simulink model "CPUTask"  (R2022b)
settings: Solver=FixedStepDiscrete  StartTime=0.0  StopTime=10.0  FixedStep=1  RelTol=1e-3
libraries: simulink x5
settings Model: Creator=sadamu  LastModifiedBy=sadamu
settings SolverCC: AlgebraicLoopSolver=TrustRegion
settings DataIOCC: ExternalInput=externalinputdata
settings OptimizationCC: DefaultParameterBehavior=Inlined  BufferReuse=off  GlobalBufferReuse=off  EnableMemcpy=off  PassReuseOutputArgsAs=Individual arguments  OptimizeDataStoreBuffers=off  BusAssignmentInplaceUpdate=off  OptimizationLevel=level0  OptimizationPriority=Speed  EfficientTunableParamExpr=on
settings DebuggingCC: ParameterTunabilityLossMsg=error  UnconnectedInputMsg=warning  UnconnectedOutputMsg=warning  UnconnectedLineMsg=warning  SFMachineParentedDataDiag=warning
settings ModelReferenceCC: EnableRefExpFcnMdlSchedulingChecks=on
settings SFSimCC: MATLABDynamicMemAlloc=off
settings RTWCC: Description=Embedded Coder  SystemTargetFile=ert.tlc  GenCodeOnly=on  TemplateMakefile=ert_default_tmf
settings CodeAppCC: GenerateComments=off  IgnoreCustomStorageClasses=off  OperatorAnnotations=on  SimulinkDataObjDesc=on  SFDataObjDesc=on  SimulinkBlockComments=off
settings ERTTargetCC: TargetLangStandard=C99 (ISO)  GenerateSampleERTMain=on  SuppressErrorStatus=on  CodeInterfacePackaging=Reusable function  InlinedParameterPlacement=NonHierarchical  MultiInstanceErrorCode=None  ERTCustomFileTemplate=example_file_process.tlc  ConvertIfToSwitch=off
settings ConfigComp: DVMaxProcessTime=3600  DVMaxTestCaseSteps=30  DVTestSuiteOptimization=Auto  DVDetectOutOfBounds=on  DVProvingStrategy=FindViolation  DVMaxViolationSteps=200000  DVModelReferenceHarness=on

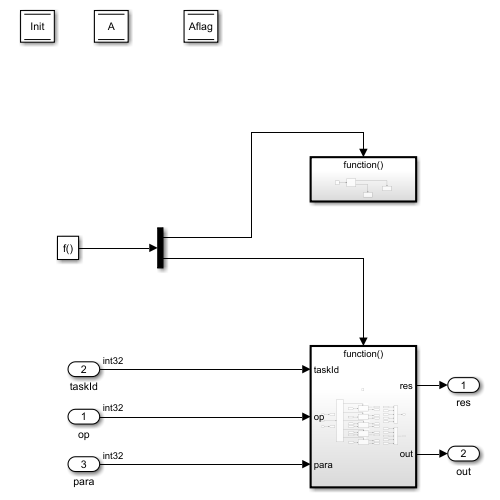
[thumbnail: Simulink's stored preview of the top-level diagram]
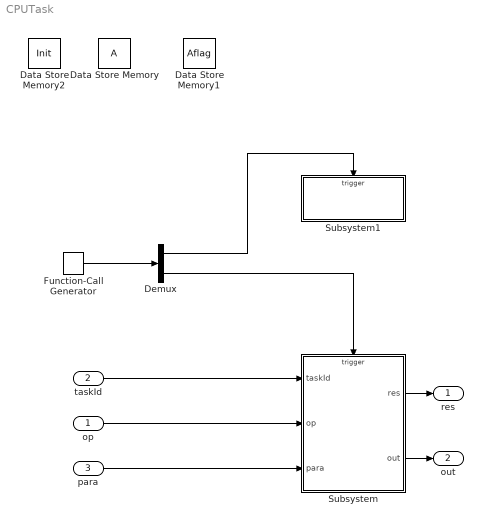
== system CPUTask ==
  op : Inport  OutDataTypeStr=int32
  taskId : Inport  Port=2  OutDataTypeStr=int32
  para : Inport  Port=3  OutDataTypeStr=int32
  Data Store Memory : DataStoreMemory  ReadBeforeWriteMsg=warning  WriteAfterWriteMsg=warning  WriteAfterReadMsg=warning  ShowAdditionalParam=off  OutDataTypeStr=int32  Dimensions=16
  Data Store Memory1 : DataStoreMemory  DataStoreName=Aflag  ReadBeforeWriteMsg=warning  WriteAfterWriteMsg=warning  WriteAfterReadMsg=warning  ShowAdditionalParam=off  OutDataTypeStr=int8  Dimensions=16
  Data Store Memory2 : DataStoreMemory  DataStoreName=Init  ReadBeforeWriteMsg=warning  WriteAfterWriteMsg=warning  WriteAfterReadMsg=warning  ShowAdditionalParam=off  OutDataTypeStr=int8  Dimensions=1
  Demux : Demux  Outputs=2
  Function-Call Generator : simulink/Ports & Subsystems/Function-Call Generator  sample_time=1  numberOfIterations=1  DisallowWideOutput=off
  Subsystem : Subsystem
  Subsystem1 : Subsystem
  res : Outport
  out : Outport  Port=2
  wires:
  taskId/1 -> Subsystem/1(taskId)
  op/1 -> Subsystem/2(op)
  para/1 -> Subsystem/3(para)
  Subsystem/1(res) -> res/1
  Subsystem/2(out) -> out/1
  Demux/1 -> Subsystem1/Trigger
  Function-Call Generator/1 -> Demux/1
  Demux/2 -> Subsystem/Trigger

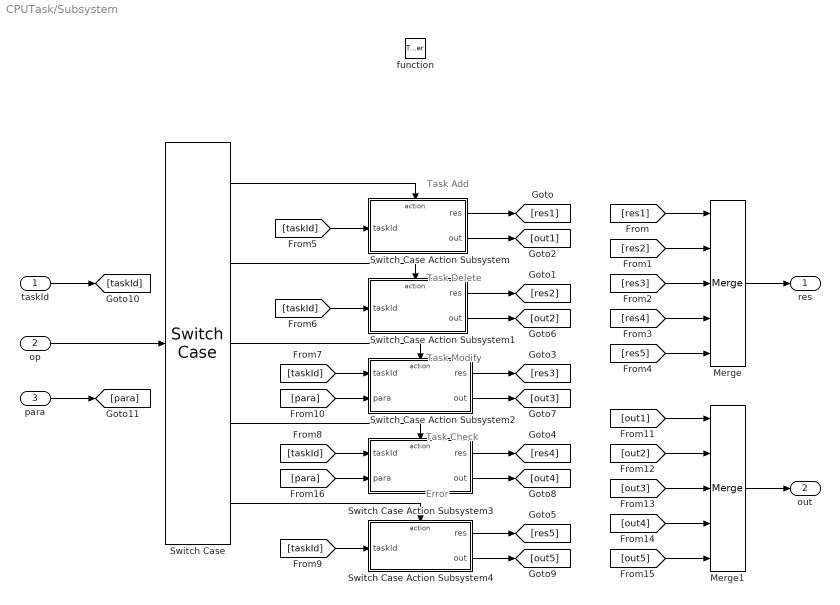
== system CPUTask/Subsystem ==
  note: Task Add
  note: Task Delete
  note: Task Modify
  note: Task Check
  note: Error
  taskId : Inport
  op : Inport  Port=2
  para : Inport  Port=3
  function : TriggerPort  TriggerType=function-call  VariantControl=Variant
  Merge : Merge  Inputs=5
  Merge1 : Merge  Inputs=5
  Switch Case : SwitchCase  CaseConditions={1,2,3,4}
  Switch Case Action Subsystem : Subsystem  TreatAsAtomicUnit=on
  Switch Case Action Subsystem1 : Subsystem  TreatAsAtomicUnit=on
  Switch Case Action Subsystem2 : Subsystem  TreatAsAtomicUnit=on
  Switch Case Action Subsystem3 : Subsystem  TreatAsAtomicUnit=on
  Switch Case Action Subsystem4 : Subsystem  TreatAsAtomicUnit=on
  res : Outport
  out : Outport  Port=2
  wires:
  Merge/1 -> res/1
  op/1 -> Switch Case/1
  Switch Case Action Subsystem/1(res) -> [res1]
  Merge1/1 -> out/1
  [res1] -> Merge/1
  [res2] -> Merge/2
  [res3] -> Merge/3
  [res4] -> Merge/4
  [res5] -> Merge/5
  Switch Case Action Subsystem1/1(res) -> [res2]
  Switch Case Action Subsystem/2(out) -> [out1]
  Switch Case Action Subsystem2/1(res) -> [res3]
  Switch Case Action Subsystem3/1(res) -> [res4]
  Switch Case Action Subsystem4/1(res) -> [res5]
  Switch Case Action Subsystem1/2(out) -> [out2]
  Switch Case Action Subsystem2/2(out) -> [out3]
  Switch Case Action Subsystem3/2(out) -> [out4]
  Switch Case Action Subsystem4/2(out) -> [out5]
  taskId/1 -> [taskId]
  para/1 -> [para]
  Switch Case/1 -> Switch Case Action Subsystem/Action
  Switch Case/2 -> Switch Case Action Subsystem1/Action
  Switch Case/3 -> Switch Case Action Subsystem2/Action
  Switch Case/4 -> Switch Case Action Subsystem3/Action
  Switch Case/5 -> Switch Case Action Subsystem4/Action
  [taskId] -> Switch Case Action Subsystem/1(taskId)
  [taskId] -> Switch Case Action Subsystem1/1(taskId)
  [taskId] -> Switch Case Action Subsystem2/1(taskId)
  [taskId] -> Switch Case Action Subsystem3/1(taskId)
  [taskId] -> Switch Case Action Subsystem4/1(taskId)
  [para] -> Switch Case Action Subsystem2/2(para)
  [out1] -> Merge1/1
  [out2] -> Merge1/2
  [out3] -> Merge1/3
  [out4] -> Merge1/4
  [out5] -> Merge1/5
  [para] -> Switch Case Action Subsystem3/2(para)

== system CPUTask/Subsystem1 ==
  function : TriggerPort  TriggerType=function-call  VariantControl=Variant
  Data Store Read : DataStoreRead  DataStoreName=Init  IndexOptions=Index vector (dialog)  Indices=1  OutputSizes=1
  If : If
  If Action Subsystem : Subsystem  TreatAsAtomicUnit=on
  If Action Subsystem1 : Subsystem  TreatAsAtomicUnit=on
  wires:
  Data Store Read/1 -> If/1
  If/2 -> If Action Subsystem/Action
  If/1 -> If Action Subsystem1/Action

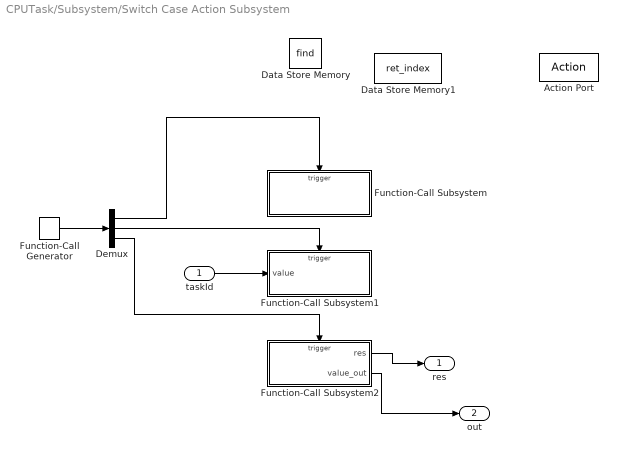
== system CPUTask/Subsystem/Switch Case Action Subsystem ==
  taskId : Inport
  Action Port : ActionPort  ActionPortLabel=case [ 1 ]:
  Data Store Memory : DataStoreMemory  DataStoreName=find  ReadBeforeWriteMsg=warning  WriteAfterWriteMsg=warning  WriteAfterReadMsg=warning  ShowAdditionalParam=off  OutDataTypeStr=int32
  Data Store Memory1 : DataStoreMemory  DataStoreName=ret_index  ReadBeforeWriteMsg=warning  WriteAfterWriteMsg=warning  WriteAfterReadMsg=warning  ShowAdditionalParam=off  OutDataTypeStr=int32
  Demux : Demux  Outputs=3
  Function-Call Generator : simulink/Ports & Subsystems/Function-Call Generator  sample_time=-1  numberOfIterations=1  DisallowWideOutput=off
  Function-Call Subsystem : Subsystem  TreatAsAtomicUnit=on
  Function-Call Subsystem1 : Subsystem  TreatAsAtomicUnit=on
  Function-Call Subsystem2 : Subsystem  TreatAsAtomicUnit=on
  res : Outport
  out : Outport  Port=2
  wires:
  taskId/1 -> Function-Call Subsystem1/1(value)
  Function-Call Generator/1 -> Demux/1
  Demux/1 -> Function-Call Subsystem/Trigger
  Demux/2 -> Function-Call Subsystem1/Trigger
  Demux/3 -> Function-Call Subsystem2/Trigger
  Function-Call Subsystem2/2(value_out) -> out/1
  Function-Call Subsystem2/1(res) -> res/1

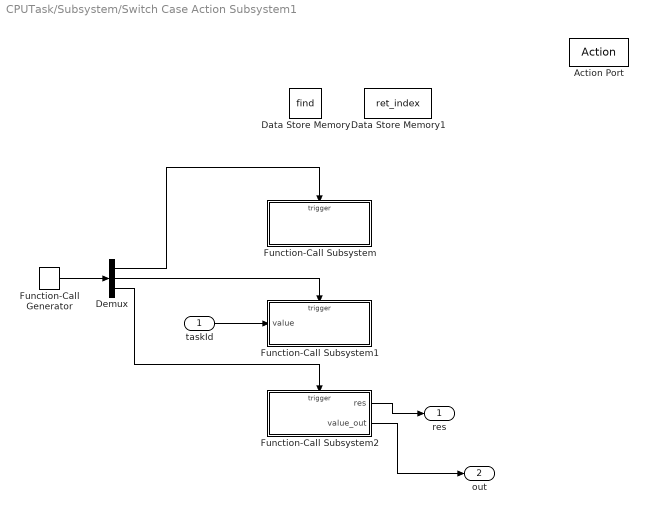
== system CPUTask/Subsystem/Switch Case Action Subsystem1 ==
  taskId : Inport
  Action Port : ActionPort  ActionPortLabel=case [ 2 ]:
  Data Store Memory : DataStoreMemory  DataStoreName=find  ReadBeforeWriteMsg=warning  WriteAfterWriteMsg=warning  WriteAfterReadMsg=warning  ShowAdditionalParam=off  OutDataTypeStr=int32
  Data Store Memory1 : DataStoreMemory  DataStoreName=ret_index  ReadBeforeWriteMsg=warning  WriteAfterWriteMsg=warning  WriteAfterReadMsg=warning  ShowAdditionalParam=off  OutDataTypeStr=int32
  Demux : Demux  Outputs=3
  Function-Call Generator : simulink/Ports & Subsystems/Function-Call Generator  sample_time=-1  numberOfIterations=1  DisallowWideOutput=off
  Function-Call Subsystem : Subsystem  TreatAsAtomicUnit=on
  Function-Call Subsystem1 : Subsystem  TreatAsAtomicUnit=on
  Function-Call Subsystem2 : Subsystem  TreatAsAtomicUnit=on
  res : Outport
  out : Outport  Port=2
  wires:
  Function-Call Subsystem2/1(res) -> res/1
  taskId/1 -> Function-Call Subsystem1/1(value)
  Demux/2 -> Function-Call Subsystem1/Trigger
  Demux/1 -> Function-Call Subsystem/Trigger
  Function-Call Generator/1 -> Demux/1
  Function-Call Subsystem2/2(value_out) -> out/1
  Demux/3 -> Function-Call Subsystem2/Trigger

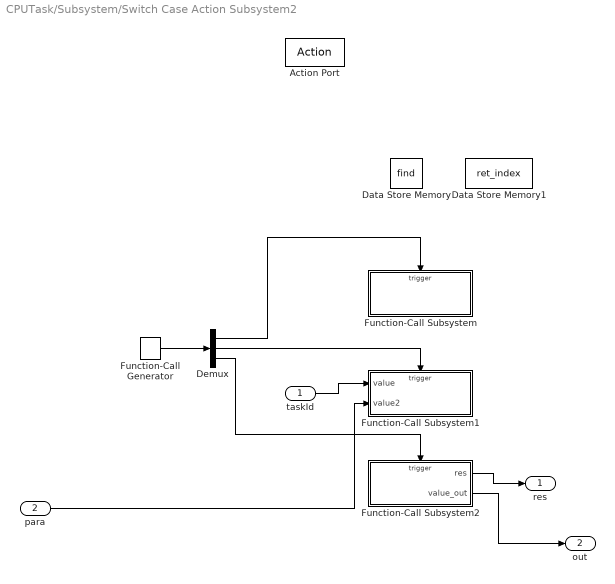
== system CPUTask/Subsystem/Switch Case Action Subsystem2 ==
  taskId : Inport
  para : Inport  Port=2
  Action Port : ActionPort  ActionPortLabel=case [ 3 ]:
  Data Store Memory : DataStoreMemory  DataStoreName=find  ReadBeforeWriteMsg=warning  WriteAfterWriteMsg=warning  WriteAfterReadMsg=warning  ShowAdditionalParam=off  OutDataTypeStr=int32
  Data Store Memory1 : DataStoreMemory  DataStoreName=ret_index  ReadBeforeWriteMsg=warning  WriteAfterWriteMsg=warning  WriteAfterReadMsg=warning  ShowAdditionalParam=off  OutDataTypeStr=int32
  Demux : Demux  Outputs=3
  Function-Call Generator : simulink/Ports & Subsystems/Function-Call Generator  sample_time=-1  numberOfIterations=1  DisallowWideOutput=off
  Function-Call Subsystem : Subsystem  TreatAsAtomicUnit=on
  Function-Call Subsystem1 : Subsystem  TreatAsAtomicUnit=on
  Function-Call Subsystem2 : Subsystem  TreatAsAtomicUnit=on
  res : Outport
  out : Outport  Port=2
  wires:
  Demux/2 -> Function-Call Subsystem1/Trigger
  Function-Call Generator/1 -> Demux/1
  Demux/3 -> Function-Call Subsystem2/Trigger
  Demux/1 -> Function-Call Subsystem/Trigger
  taskId/1 -> Function-Call Subsystem1/1(value)
  Function-Call Subsystem2/1(res) -> res/1
  Function-Call Subsystem2/2(value_out) -> out/1
  para/1 -> Function-Call Subsystem1/2(value2)

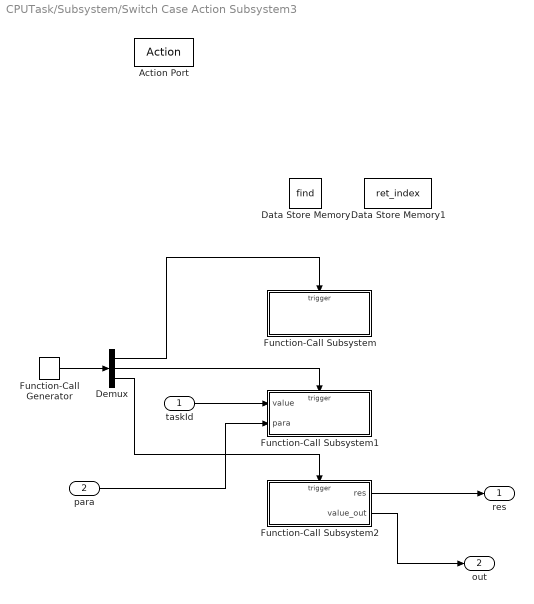
== system CPUTask/Subsystem/Switch Case Action Subsystem3 ==
  taskId : Inport
  para : Inport  Port=2
  Action Port : ActionPort  ActionPortLabel=case [ 4 ]:
  Data Store Memory : DataStoreMemory  DataStoreName=find  ReadBeforeWriteMsg=warning  WriteAfterWriteMsg=warning  WriteAfterReadMsg=warning  ShowAdditionalParam=off  OutDataTypeStr=int32
  Data Store Memory1 : DataStoreMemory  DataStoreName=ret_index  ReadBeforeWriteMsg=warning  WriteAfterWriteMsg=warning  WriteAfterReadMsg=warning  ShowAdditionalParam=off  OutDataTypeStr=int32
  Demux : Demux  Outputs=3
  Function-Call Generator : simulink/Ports & Subsystems/Function-Call Generator  sample_time=-1  numberOfIterations=1  DisallowWideOutput=off
  Function-Call Subsystem : Subsystem  TreatAsAtomicUnit=on
  Function-Call Subsystem1 : Subsystem  TreatAsAtomicUnit=on
  Function-Call Subsystem2 : Subsystem  TreatAsAtomicUnit=on
  res : Outport
  out : Outport  Port=2
  wires:
  Function-Call Generator/1 -> Demux/1
  taskId/1 -> Function-Call Subsystem1/1(value)
  Demux/3 -> Function-Call Subsystem2/Trigger
  Function-Call Subsystem2/1(res) -> res/1
  Function-Call Subsystem2/2(value_out) -> out/1
  Demux/1 -> Function-Call Subsystem/Trigger
  Demux/2 -> Function-Call Subsystem1/Trigger
  para/1 -> Function-Call Subsystem1/2(para)

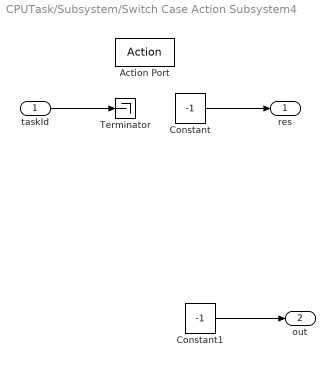
== system CPUTask/Subsystem/Switch Case Action Subsystem4 ==
  taskId : Inport
  Action Port : ActionPort  ActionPortLabel=default:
  Constant : Constant  Value=-1  OutDataTypeStr=int32
  Constant1 : Constant  Value=-1  OutDataTypeStr=int32
  Terminator : Terminator
  res : Outport
  out : Outport  Port=2
  wires:
  taskId/1 -> Terminator/1
  Constant/1 -> res/1
  Constant1/1 -> out/1

== system CPUTask/Subsystem1/If Action Subsystem ==
  Action Port : ActionPort  ActionPortLabel=else
  Constant : Constant  Value=0  OutDataTypeStr=int8
  Constant1 : Constant  OutDataTypeStr=int8
  Data Store Write : DataStoreWrite  DataStoreName=Init  IndexOptions=Index vector (dialog)  Indices=1  OutputSizes=1
  For Iterator Subsystem : Subsystem  TreatAsAtomicUnit=on
  wires:
  Constant/1 -> For Iterator Subsystem/1(In1)
  Constant1/1 -> Data Store Write/1

== system CPUTask/Subsystem1/If Action Subsystem1 ==
  Action Port : ActionPort  ActionPortLabel=if(u1 > 0)

== system CPUTask/Subsystem/Switch Case Action Subsystem/Function-Call Subsystem ==
  function : TriggerPort  TriggerType=function-call  VariantControl=Variant
  Constant : Constant  Value=0  OutDataTypeStr=int32
  Constant1 : Constant  Value=-1  OutDataTypeStr=int32
  Data Store Write : DataStoreWrite  DataStoreName=ret_index  IndexOptions=Index vector (dialog)  Indices=1  OutputSizes=1
  Data Store Write1 : DataStoreWrite  DataStoreName=find  IndexOptions=Index vector (dialog)  Indices=1  OutputSizes=1
  wires:
  Constant/1 -> Data Store Write1/1
  Constant1/1 -> Data Store Write/1

== system CPUTask/Subsystem/Switch Case Action Subsystem/Function-Call Subsystem1 ==
  value : Inport
  function : TriggerPort  TriggerType=function-call  VariantControl=Variant
  For Iterator Subsystem : Subsystem  TreatAsAtomicUnit=on
  wires:
  value/1 -> For Iterator Subsystem/1(value)

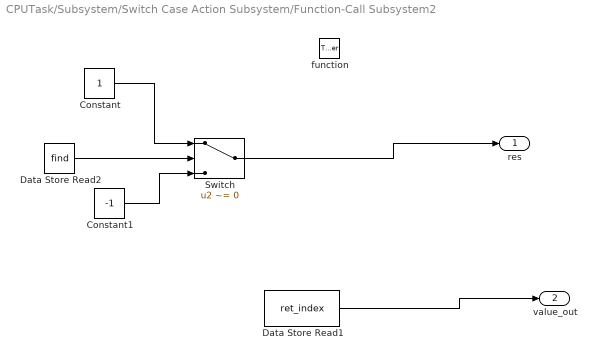
== system CPUTask/Subsystem/Switch Case Action Subsystem/Function-Call Subsystem2 ==
  function : TriggerPort  TriggerType=function-call  VariantControl=Variant
  Constant : Constant  OutDataTypeStr=int32
  Constant1 : Constant  Value=-1  OutDataTypeStr=int32
  Data Store Read1 : DataStoreRead  DataStoreName=ret_index  IndexOptions=Index vector (dialog)  Indices=1  OutputSizes=1
  Data Store Read2 : DataStoreRead  DataStoreName=find  IndexOptions=Index vector (dialog)  Indices=1  OutputSizes=1
  Switch : Switch  Criteria=u2 ~= 0  SaturateOnIntegerOverflow=off  InputSameDT=off
  res : Outport
  value_out : Outport  Port=2
  wires:
  Switch/1 -> res/1
  Data Store Read1/1 -> value_out/1
  Data Store Read2/1 -> Switch/2
  Constant1/1 -> Switch/3
  Constant/1 -> Switch/1

== system CPUTask/Subsystem/Switch Case Action Subsystem1/Function-Call Subsystem ==
  function : TriggerPort  TriggerType=function-call  VariantControl=Variant
  Constant : Constant  Value=0  OutDataTypeStr=int32
  Constant1 : Constant  Value=-1  OutDataTypeStr=int32
  Data Store Write : DataStoreWrite  DataStoreName=ret_index  IndexOptions=Index vector (dialog)  Indices=1  OutputSizes=1
  Data Store Write1 : DataStoreWrite  DataStoreName=find  IndexOptions=Index vector (dialog)  Indices=1  OutputSizes=1
  wires:
  Constant/1 -> Data Store Write1/1
  Constant1/1 -> Data Store Write/1

== system CPUTask/Subsystem/Switch Case Action Subsystem1/Function-Call Subsystem1 ==
  value : Inport
  function : TriggerPort  TriggerType=function-call  VariantControl=Variant
  For Iterator Subsystem : Subsystem  TreatAsAtomicUnit=on
  wires:
  value/1 -> For Iterator Subsystem/1(value)

== system CPUTask/Subsystem/Switch Case Action Subsystem1/Function-Call Subsystem2 ==
  function : TriggerPort  TriggerType=function-call  VariantControl=Variant
  Data Store Read : DataStoreRead  DataStoreName=find  IndexOptions=Index vector (dialog)  Indices=1  OutputSizes=1
  Data Store Read1 : DataStoreRead  DataStoreName=ret_index  IndexOptions=Index vector (dialog)  Indices=1  OutputSizes=1
  res : Outport
  value_out : Outport  Port=2
  wires:
  Data Store Read/1 -> res/1
  Data Store Read1/1 -> value_out/1

== system CPUTask/Subsystem/Switch Case Action Subsystem2/Function-Call Subsystem ==
  function : TriggerPort  TriggerType=function-call  VariantControl=Variant
  Constant : Constant  Value=0  OutDataTypeStr=int32
  Constant1 : Constant  Value=-1  OutDataTypeStr=int32
  Data Store Write : DataStoreWrite  DataStoreName=ret_index  IndexOptions=Index vector (dialog)  Indices=1  OutputSizes=1
  Data Store Write1 : DataStoreWrite  DataStoreName=find  IndexOptions=Index vector (dialog)  Indices=1  OutputSizes=1
  wires:
  Constant/1 -> Data Store Write1/1
  Constant1/1 -> Data Store Write/1

== system CPUTask/Subsystem/Switch Case Action Subsystem2/Function-Call Subsystem1 ==
  value : Inport
  value2 : Inport  Port=2
  function : TriggerPort  TriggerType=function-call  VariantControl=Variant
  For Iterator Subsystem : Subsystem  TreatAsAtomicUnit=on
  wires:
  value/1 -> For Iterator Subsystem/1(value)
  value2/1 -> For Iterator Subsystem/2(value2)

== system CPUTask/Subsystem/Switch Case Action Subsystem2/Function-Call Subsystem2 ==
  function : TriggerPort  TriggerType=function-call  VariantControl=Variant
  Data Store Read : DataStoreRead  DataStoreName=find  IndexOptions=Index vector (dialog)  Indices=1  OutputSizes=1
  Data Store Read1 : DataStoreRead  DataStoreName=ret_index  IndexOptions=Index vector (dialog)  Indices=1  OutputSizes=1
  res : Outport
  value_out : Outport  Port=2
  wires:
  Data Store Read/1 -> res/1
  Data Store Read1/1 -> value_out/1

== system CPUTask/Subsystem/Switch Case Action Subsystem3/Function-Call Subsystem ==
  function : TriggerPort  TriggerType=function-call  VariantControl=Variant
  Constant : Constant  Value=0  OutDataTypeStr=int32
  Constant1 : Constant  Value=-1  OutDataTypeStr=int32
  Data Store Write : DataStoreWrite  DataStoreName=ret_index  IndexOptions=Index vector (dialog)  Indices=1  OutputSizes=1
  Data Store Write1 : DataStoreWrite  DataStoreName=find  IndexOptions=Index vector (dialog)  Indices=1  OutputSizes=1
  wires:
  Constant/1 -> Data Store Write1/1
  Constant1/1 -> Data Store Write/1

== system CPUTask/Subsystem/Switch Case Action Subsystem3/Function-Call Subsystem1 ==
  value : Inport
  para : Inport  Port=2
  function : TriggerPort  TriggerType=function-call  VariantControl=Variant
  For Iterator Subsystem : Subsystem  TreatAsAtomicUnit=on
  wires:
  value/1 -> For Iterator Subsystem/1(value)

== system CPUTask/Subsystem/Switch Case Action Subsystem3/Function-Call Subsystem2 ==
  function : TriggerPort  TriggerType=function-call  VariantControl=Variant
  Data Store Read : DataStoreRead  DataStoreName=find  IndexOptions=Index vector (dialog)  Indices=1  OutputSizes=1
  Data Store Read1 : DataStoreRead  DataStoreName=ret_index  IndexOptions=Index vector (dialog)  Indices=1  OutputSizes=1
  res : Outport
  value_out : Outport  Port=2
  wires:
  Data Store Read/1 -> res/1
  Data Store Read1/1 -> value_out/1

== system CPUTask/Subsystem1/If Action Subsystem/For Iterator Subsystem ==
  In1 : Inport
  Assignment : Assignment  IndexMode=Zero-based  DiagnosticForDimensions=Warning  IndexOptions=Index vector (port)  Indices=1  OutputSizes=1
  Data Store Read : DataStoreRead  DataStoreName=Aflag  IndexOptions=Index vector (dialog)  Indices=1  OutputSizes=1
  Data Store Write : DataStoreWrite  DataStoreName=Aflag  IndexOptions=Index vector (dialog)  Indices=1  OutputSizes=1
  For Iterator : ForIterator  IterationLimit=16  IndexMode=Zero-based
  wires:
  In1/1 -> Assignment/2
  For Iterator/1 -> Assignment/3
  Data Store Read/1 -> Assignment/1
  Assignment/1 -> Data Store Write/1

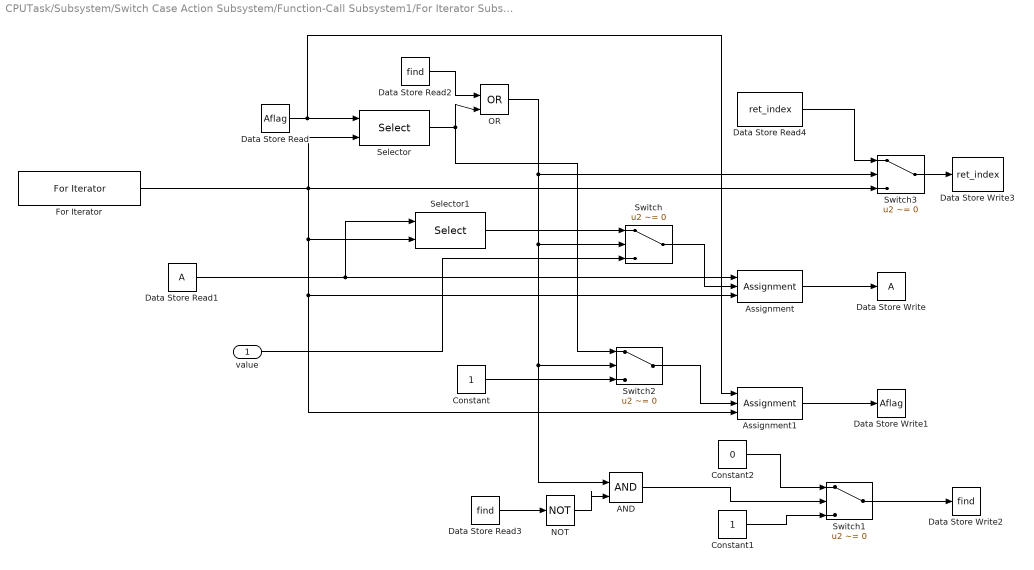
== system CPUTask/Subsystem/Switch Case Action Subsystem/Function-Call Subsystem1/For Iterator Subsystem ==
  value : Inport
  AND : Logic  IconShape=distinctive  AllPortsSameDT=off  OutDataTypeStr=boolean
  Assignment : Assignment  IndexMode=Zero-based  DiagnosticForDimensions=Warning  IndexOptions=Index vector (port)  Indices=1  OutputSizes=1
  Assignment1 : Assignment  IndexMode=Zero-based  DiagnosticForDimensions=Warning  IndexOptions=Index vector (port)  Indices=1  OutputSizes=1
  Constant : Constant  OutDataTypeStr=int8
  Constant1 : Constant  OutDataTypeStr=int32
  Constant2 : Constant  Value=0  OutDataTypeStr=int32
  Data Store Read : DataStoreRead  DataStoreName=Aflag  IndexOptions=Index vector (dialog)  Indices=1  OutputSizes=1
  Data Store Read1 : DataStoreRead  IndexOptions=Index vector (dialog)  Indices=1  OutputSizes=1
  Data Store Read2 : DataStoreRead  DataStoreName=find  IndexOptions=Index vector (dialog)  Indices=1  OutputSizes=1
  Data Store Read3 : DataStoreRead  DataStoreName=find  IndexOptions=Index vector (dialog)  Indices=1  OutputSizes=1
  Data Store Read4 : DataStoreRead  DataStoreName=ret_index  IndexOptions=Index vector (dialog)  Indices=1  OutputSizes=1
  Data Store Write : DataStoreWrite  IndexOptions=Index vector (dialog)  Indices=1  OutputSizes=1
  Data Store Write1 : DataStoreWrite  DataStoreName=Aflag  IndexOptions=Index vector (dialog)  Indices=1  OutputSizes=1
  Data Store Write2 : DataStoreWrite  DataStoreName=find  IndexOptions=Index vector (dialog)  Indices=1  OutputSizes=1
  Data Store Write3 : DataStoreWrite  DataStoreName=ret_index  IndexOptions=Index vector (dialog)  Indices=1  OutputSizes=1
  For Iterator : ForIterator  IterationLimit=16  IndexMode=Zero-based
  NOT : Logic  Operator=NOT  IconShape=distinctive  AllPortsSameDT=off  OutDataTypeStr=boolean
  OR : Logic  Operator=OR  IconShape=distinctive  AllPortsSameDT=off  OutDataTypeStr=boolean
  Selector : Selector  IndexMode=Zero-based  InputPortWidth=16  IndexOptions=Index vector (port)  Indices=[1 3]  OutputSizes=1
  Selector1 : Selector  IndexMode=Zero-based  InputPortWidth=16  IndexOptions=Index vector (port)  Indices=[1 3]  OutputSizes=1
  Switch{,1..3} (4 alike) : Switch  Criteria=u2 ~= 0  SaturateOnIntegerOverflow=off  InputSameDT=off
  wires:
  value/1 -> Switch/3
  Data Store Read/1 -> Assignment1/1, Selector/1
  Selector/1 -> Switch2/1, OR/2
  Data Store Read1/1 -> Selector1/1, Assignment/1
  Selector1/1 -> Switch/1
  Switch/1 -> Assignment/2
  Assignment/1 -> Data Store Write/1
  Data Store Read2/1 -> OR/1
  Switch1/1 -> Data Store Write2/1
  Constant1/1 -> Switch1/3
  Constant2/1 -> Switch1/1
  Data Store Read3/1 -> NOT/1
  AND/1 -> Switch1/2
  NOT/1 -> AND/2
  Constant/1 -> Switch2/3
  Switch2/1 -> Assignment1/2
  Assignment1/1 -> Data Store Write1/1
  Data Store Read4/1 -> Switch3/1
  Switch3/1 -> Data Store Write3/1
  OR/1 -> Switch3/2, AND/1, Switch2/2, Switch/2
  For Iterator/1 -> Assignment1/3, Assignment/3, Selector1/2, Selector/2, Switch3/3

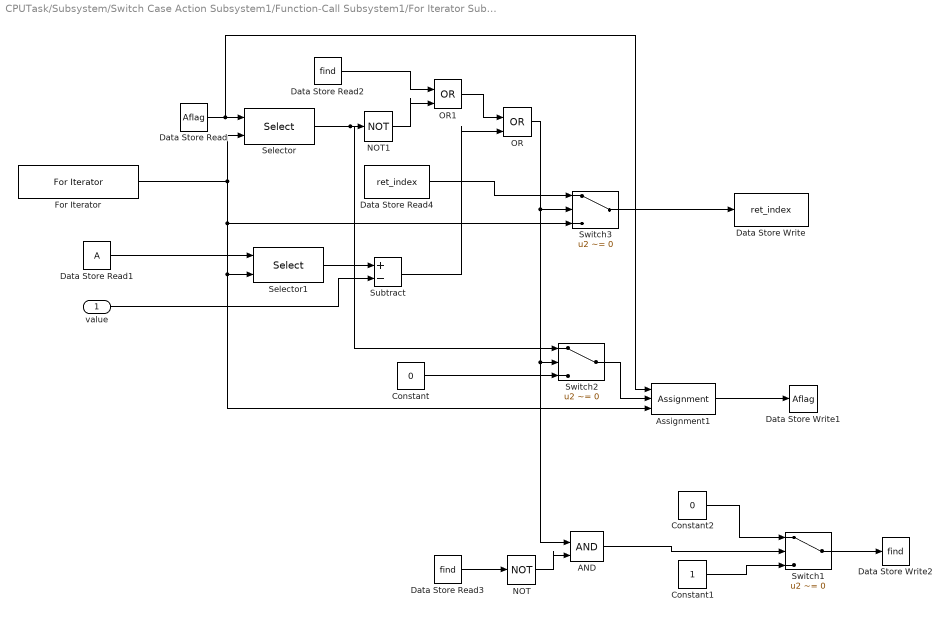
== system CPUTask/Subsystem/Switch Case Action Subsystem1/Function-Call Subsystem1/For Iterator Subsystem ==
  value : Inport
  AND : Logic  IconShape=distinctive  AllPortsSameDT=off  OutDataTypeStr=boolean
  Assignment1 : Assignment  IndexMode=Zero-based  DiagnosticForDimensions=Warning  IndexOptions=Index vector (port)  Indices=1  OutputSizes=1
  Constant : Constant  Value=0  OutDataTypeStr=int8
  Constant1 : Constant  OutDataTypeStr=int32
  Constant2 : Constant  Value=0  OutDataTypeStr=int32
  Data Store Read : DataStoreRead  DataStoreName=Aflag  IndexOptions=Index vector (dialog)  Indices=1  OutputSizes=1
  Data Store Read1 : DataStoreRead  IndexOptions=Index vector (dialog)  Indices=1  OutputSizes=1
  Data Store Read2 : DataStoreRead  DataStoreName=find  IndexOptions=Index vector (dialog)  Indices=1  OutputSizes=1
  Data Store Read3 : DataStoreRead  DataStoreName=find  IndexOptions=Index vector (dialog)  Indices=1  OutputSizes=1
  Data Store Read4 : DataStoreRead  DataStoreName=ret_index  IndexOptions=Index vector (dialog)  Indices=1  OutputSizes=1
  Data Store Write : DataStoreWrite  DataStoreName=ret_index  IndexOptions=Index vector (dialog)  Indices=1  OutputSizes=1
  Data Store Write1 : DataStoreWrite  DataStoreName=Aflag  IndexOptions=Index vector (dialog)  Indices=1  OutputSizes=1
  Data Store Write2 : DataStoreWrite  DataStoreName=find  IndexOptions=Index vector (dialog)  Indices=1  OutputSizes=1
  For Iterator : ForIterator  IterationLimit=16  IndexMode=Zero-based
  NOT : Logic  Operator=NOT  IconShape=distinctive  AllPortsSameDT=off  OutDataTypeStr=boolean
  NOT1 : Logic  Operator=NOT  IconShape=distinctive  AllPortsSameDT=off  OutDataTypeStr=boolean
  OR : Logic  Operator=OR  IconShape=distinctive  AllPortsSameDT=off  OutDataTypeStr=boolean
  OR1 : Logic  Operator=OR  IconShape=distinctive  AllPortsSameDT=off  OutDataTypeStr=boolean
  Selector : Selector  IndexMode=Zero-based  InputPortWidth=16  IndexOptions=Index vector (port)  Indices=[1 3]  OutputSizes=1
  Selector1 : Selector  IndexMode=Zero-based  InputPortWidth=16  IndexOptions=Index vector (port)  Indices=[1 3]  OutputSizes=1
  Subtract : Sum  Inputs=+-
  Switch1 : Switch  Criteria=u2 ~= 0  SaturateOnIntegerOverflow=off  InputSameDT=off
  Switch2 : Switch  Criteria=u2 ~= 0  SaturateOnIntegerOverflow=off  InputSameDT=off
  Switch3 : Switch  Criteria=u2 ~= 0  SaturateOnIntegerOverflow=off  InputSameDT=off
  wires:
  For Iterator/1 -> Assignment1/3, Selector1/2, Switch3/3, Selector/2
  Data Store Read/1 -> Assignment1/1, Selector/1
  Selector/1 -> Switch2/1, NOT1/1
  Data Store Read1/1 -> Selector1/1
  OR/1 -> AND/1, Switch2/2, Switch3/2
  Data Store Read2/1 -> OR1/1
  Switch1/1 -> Data Store Write2/1
  Constant1/1 -> Switch1/3
  Constant2/1 -> Switch1/1
  Data Store Read3/1 -> NOT/1
  AND/1 -> Switch1/2
  NOT/1 -> AND/2
  Constant/1 -> Switch2/3
  Switch2/1 -> Assignment1/2
  Assignment1/1 -> Data Store Write1/1
  NOT1/1 -> OR1/2
  Selector1/1 -> Subtract/1
  value/1 -> Subtract/2
  Subtract/1 -> OR/2
  Switch3/1 -> Data Store Write/1
  Data Store Read4/1 -> Switch3/1
  OR1/1 -> OR/1

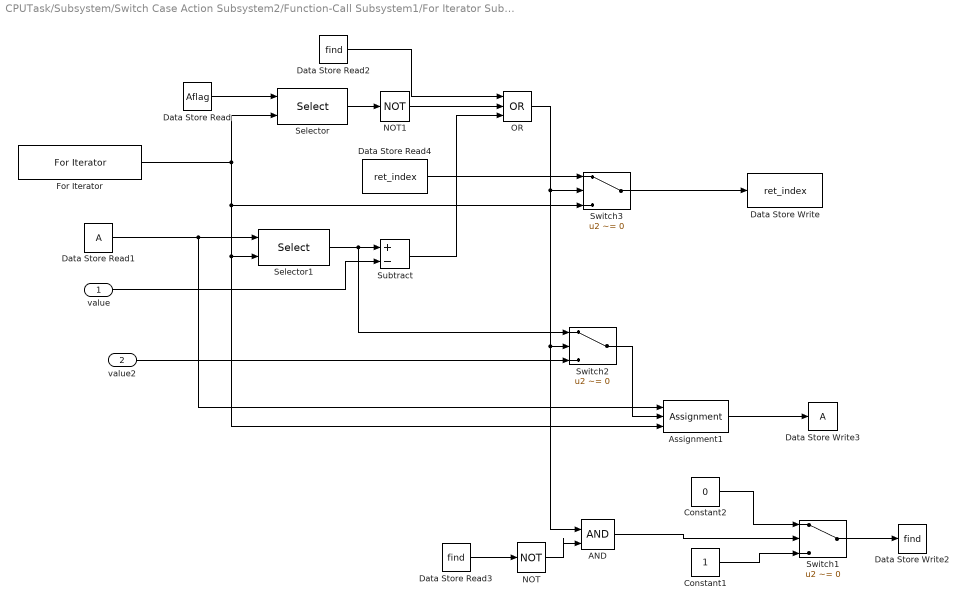
== system CPUTask/Subsystem/Switch Case Action Subsystem2/Function-Call Subsystem1/For Iterator Subsystem ==
  value : Inport
  value2 : Inport  Port=2
  AND : Logic  IconShape=distinctive  AllPortsSameDT=off  OutDataTypeStr=boolean
  Assignment1 : Assignment  IndexMode=Zero-based  DiagnosticForDimensions=Warning  IndexOptions=Index vector (port)  Indices=1  OutputSizes=1
  Constant1 : Constant  OutDataTypeStr=int32
  Constant2 : Constant  Value=0  OutDataTypeStr=int32
  Data Store Read : DataStoreRead  DataStoreName=Aflag  IndexOptions=Index vector (dialog)  Indices=1  OutputSizes=1
  Data Store Read1 : DataStoreRead  IndexOptions=Index vector (dialog)  Indices=1  OutputSizes=1
  Data Store Read2 : DataStoreRead  DataStoreName=find  IndexOptions=Index vector (dialog)  Indices=1  OutputSizes=1
  Data Store Read3 : DataStoreRead  DataStoreName=find  IndexOptions=Index vector (dialog)  Indices=1  OutputSizes=1
  Data Store Read4 : DataStoreRead  DataStoreName=ret_index  IndexOptions=Index vector (dialog)  Indices=1  OutputSizes=1
  Data Store Write : DataStoreWrite  DataStoreName=ret_index  IndexOptions=Index vector (dialog)  Indices=1  OutputSizes=1
  Data Store Write2 : DataStoreWrite  DataStoreName=find  IndexOptions=Index vector (dialog)  Indices=1  OutputSizes=1
  Data Store Write3 : DataStoreWrite  IndexOptions=Index vector (dialog)  Indices=1  OutputSizes=1
  For Iterator : ForIterator  IterationLimit=16  IndexMode=Zero-based
  NOT : Logic  Operator=NOT  IconShape=distinctive  AllPortsSameDT=off  OutDataTypeStr=boolean
  NOT1 : Logic  Operator=NOT  IconShape=distinctive  AllPortsSameDT=off  OutDataTypeStr=boolean
  OR : Logic  Operator=OR  Inputs=3  IconShape=distinctive  AllPortsSameDT=off  OutDataTypeStr=boolean
  Selector : Selector  IndexMode=Zero-based  InputPortWidth=16  IndexOptions=Index vector (port)  Indices=[1 3]  OutputSizes=1
  Selector1 : Selector  IndexMode=Zero-based  InputPortWidth=16  IndexOptions=Index vector (port)  Indices=[1 3]  OutputSizes=1
  Subtract : Sum  Inputs=+-
  Switch1 : Switch  Criteria=u2 ~= 0  SaturateOnIntegerOverflow=off  InputSameDT=off
  Switch2 : Switch  Criteria=u2 ~= 0  SaturateOnIntegerOverflow=off  InputSameDT=off
  Switch3 : Switch  Criteria=u2 ~= 0  SaturateOnIntegerOverflow=off  InputSameDT=off
  wires:
  For Iterator/1 -> Assignment1/3, Selector1/2, Switch3/3, Selector/2
  Data Store Read/1 -> Selector/1
  Selector/1 -> NOT1/1
  Data Store Read1/1 -> Assignment1/1, Selector1/1
  OR/1 -> AND/1, Switch2/2, Switch3/2
  Data Store Read2/1 -> OR/1
  Switch1/1 -> Data Store Write2/1
  Constant1/1 -> Switch1/3
  Constant2/1 -> Switch1/1
  Data Store Read3/1 -> NOT/1
  AND/1 -> Switch1/2
  NOT/1 -> AND/2
  value2/1 -> Switch2/3
  Switch2/1 -> Assignment1/2
  Assignment1/1 -> Data Store Write3/1
  NOT1/1 -> OR/2
  Selector1/1 -> Switch2/1, Subtract/1
  value/1 -> Subtract/2
  Subtract/1 -> OR/3
  Switch3/1 -> Data Store Write/1
  Data Store Read4/1 -> Switch3/1

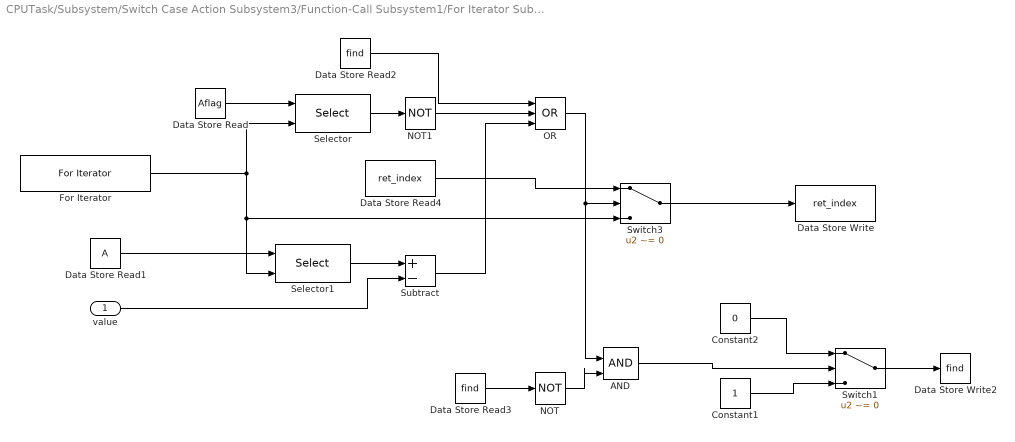
== system CPUTask/Subsystem/Switch Case Action Subsystem3/Function-Call Subsystem1/For Iterator Subsystem ==
  value : Inport
  AND : Logic  IconShape=distinctive  AllPortsSameDT=off  OutDataTypeStr=boolean
  Constant1 : Constant  OutDataTypeStr=int32
  Constant2 : Constant  Value=0  OutDataTypeStr=int32
  Data Store Read : DataStoreRead  DataStoreName=Aflag  IndexOptions=Index vector (dialog)  Indices=1  OutputSizes=1
  Data Store Read1 : DataStoreRead  IndexOptions=Index vector (dialog)  Indices=1  OutputSizes=1
  Data Store Read2 : DataStoreRead  DataStoreName=find  IndexOptions=Index vector (dialog)  Indices=1  OutputSizes=1
  Data Store Read3 : DataStoreRead  DataStoreName=find  IndexOptions=Index vector (dialog)  Indices=1  OutputSizes=1
  Data Store Read4 : DataStoreRead  DataStoreName=ret_index  IndexOptions=Index vector (dialog)  Indices=1  OutputSizes=1
  Data Store Write : DataStoreWrite  DataStoreName=ret_index  IndexOptions=Index vector (dialog)  Indices=1  OutputSizes=1
  Data Store Write2 : DataStoreWrite  DataStoreName=find  IndexOptions=Index vector (dialog)  Indices=1  OutputSizes=1
  For Iterator : ForIterator  IterationLimit=16  IndexMode=Zero-based
  NOT : Logic  Operator=NOT  IconShape=distinctive  AllPortsSameDT=off  OutDataTypeStr=boolean
  NOT1 : Logic  Operator=NOT  IconShape=distinctive  AllPortsSameDT=off  OutDataTypeStr=boolean
  OR : Logic  Operator=OR  Inputs=3  IconShape=distinctive  AllPortsSameDT=off  OutDataTypeStr=boolean
  Selector : Selector  IndexMode=Zero-based  InputPortWidth=16  IndexOptions=Index vector (port)  Indices=[1 3]  OutputSizes=1
  Selector1 : Selector  IndexMode=Zero-based  InputPortWidth=16  IndexOptions=Index vector (port)  Indices=[1 3]  OutputSizes=1
  Subtract : Sum  Inputs=+-
  Switch1 : Switch  Criteria=u2 ~= 0  SaturateOnIntegerOverflow=off  InputSameDT=off
  Switch3 : Switch  Criteria=u2 ~= 0  SaturateOnIntegerOverflow=off  InputSameDT=off
  wires:
  For Iterator/1 -> Selector1/2, Switch3/3, Selector/2
  Data Store Read/1 -> Selector/1
  Selector/1 -> NOT1/1
  Data Store Read1/1 -> Selector1/1
  OR/1 -> AND/1, Switch3/2
  Data Store Read2/1 -> OR/1
  Switch1/1 -> Data Store Write2/1
  Constant1/1 -> Switch1/3
  Constant2/1 -> Switch1/1
  Data Store Read3/1 -> NOT/1
  AND/1 -> Switch1/2
  NOT/1 -> AND/2
  NOT1/1 -> OR/2
  Selector1/1 -> Subtract/1
  value/1 -> Subtract/2
  Subtract/1 -> OR/3
  Switch3/1 -> Data Store Write/1
  Data Store Read4/1 -> Switch3/1
